simulink model "DDMRsimulink"  (R2018a)
settings: Solver=VariableStepAuto  StartTime=0.0  StopTime=tf  FixedStep=5e-3  RelTol=1e-3
InitFcn:
  | run('DDMRsimulinkParameters.m')
values from neighbouring files (symbols this model uses):
  d = 0.0445    [DDMRsimulinkParameters.m]    (also in Params.m = 1; dataSimulink.mat; p3dx_constants.m = 0.381)
  J = M*1.2e-1    (= 1.08)    [DDMRsimulinkParameters.m]    (also in Params.m = 1; dataSimulink.mat = 0.192; p3dx_constants.m = 0.2641395)
  Kb = 0.023    [DDMRsimulinkParameters.m]    (also in Params.m = 1; dataSimulink.mat = 0.029; p3dx_constants.m = 0.08)
  Kt = 0.029    [DDMRsimulinkParameters.m]    (also in Params.m = 1; dataSimulink.mat = 0.023; p3dx_constants.m = 0.01)
  L = 0.1655    [DDMRsimulinkParameters.m]    (also in Params.m = 1; dataSimulink.mat; p3dx_constants.m = 0.381)
  La = 0.66e-3    (= 0.00066)    [DDMRsimulinkParameters.m]    (also in Params.m = 1; dataSimulink.mat; p3dx_constants.m = 0.1)
  M = 9    [DDMRsimulinkParameters.m]    (also in Params.m = 1; dataSimulink.mat = 1.6; p3dx_constants.m)
  N = 38.3    [DDMRsimulinkParameters.m]    (also in Params.m = 1; dataSimulink.mat = 1; p3dx_constants.m = 38.1)
  R = 195e-3/2    (= 0.0975)    [DDMRsimulinkParameters.m]    (also in Params.m = 1; dataSimulink.mat = 0.097541; p3dx_constants.m)
  Ra = 0.71    [DDMRsimulinkParameters.m]    (also in Params.m = 1; dataSimulink.mat; p3dx_constants.m = 1)
  vaL = 5    [ExecutarSimulacoesP3DX.m]
  vaR = 12    [ExecutarSimulacoesP3DX.m]
settings Model: Creator=Egydio Tadeu  LastModifiedBy=Egydio Tadeu

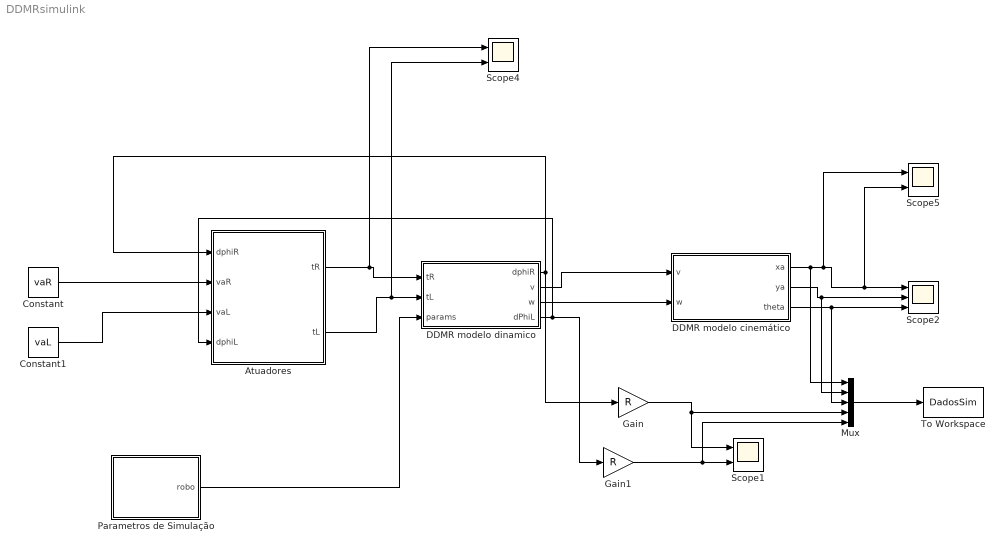
== system DDMRsimulink ==
  Atuadores : Subsystem
  Constant : Constant  Value=vaR
  Constant1 : Constant  Value=vaL
  DDMR modelo cinemático : Subsystem
  DDMR modelo dinamico : Subsystem
  Gain : Gain  Gain=R
  Gain1 : Gain  Gain=R
  Mux : Mux  Inputs=5
  Parametros de Simulação : Subsystem
  Scope1 : Scope  NumInputPorts=2
  Scope2 : Scope  NumInputPorts=3
  Scope4 : Scope  NumInputPorts=2
  Scope5 : Scope  NumInputPorts=2
  To Workspace : ToWorkspace  VariableName=DadosSim  SaveFormat=Structure With Time  SampleTime=-1
  wires:
  Parametros de Simulação/1(robo) -> DDMR modelo dinamico/3(params)
  Atuadores/1(tR) -> Scope4/1, DDMR modelo dinamico/1(tR)
  Atuadores/2(tL) -> Scope4/2, DDMR modelo dinamico/2(tL)
  DDMR modelo dinamico/4(dPhiL) -> Gain1/1, Atuadores/4(dphiL)
  DDMR modelo dinamico/1(dphiR) -> Atuadores/1(dphiR), Gain/1
  Gain1/1 -> Mux/5, Scope1/2
  Gain/1 -> Mux/4, Scope1/1
  DDMR modelo dinamico/2(v) -> DDMR modelo cinemático/1(v)
  DDMR modelo dinamico/3(w) -> DDMR modelo cinemático/2(w)
  DDMR modelo cinemático/2(ya) -> Mux/2, Scope2/2
  DDMR modelo cinemático/3(theta) -> Mux/3, Scope2/3
  DDMR modelo cinemático/1(xa) -> Mux/1, Scope5/1, Scope5/2, Scope2/1
  Constant/1 -> Atuadores/2(vaR)
  Constant1/1 -> Atuadores/3(vaL)
  Mux/1 -> To Workspace/1

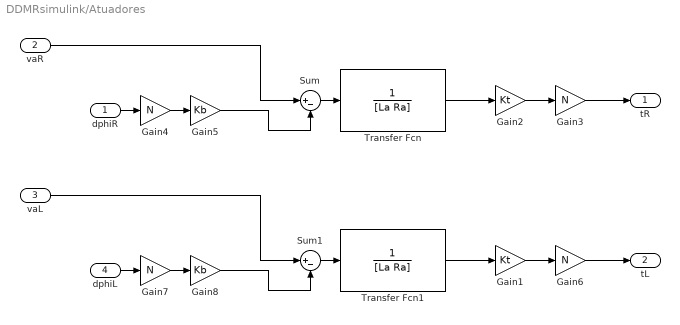
== system DDMRsimulink/Atuadores ==
  dphiR : Inport
  vaR : Inport  Port=2
  vaL : Inport  Port=3
  dphiL : Inport  Port=4
  Gain1 : Gain  Gain=Kt
  Gain2 : Gain  Gain=Kt
  Gain{3..4,6..7} (4 alike) : Gain  Gain=N
  Gain5 : Gain  Gain=Kb
  Gain8 : Gain  Gain=Kb
  Sum : Sum  Inputs=|+-
  Sum1 : Sum  Inputs=|+-
  Transfer Fcn : TransferFcn  Denominator=[La Ra]
  Transfer Fcn1 : TransferFcn  Denominator=[La Ra]
  tR : Outport
  tL : Outport  Port=2
  wires:
  Gain3/1 -> tR/1
  Transfer Fcn/1 -> Gain2/1
  Gain2/1 -> Gain3/1
  vaR/1 -> Sum/1
  Gain4/1 -> Gain5/1
  dphiR/1 -> Gain4/1
  Gain5/1 -> Sum/2
  dphiL/1 -> Gain7/1
  Gain6/1 -> tL/1
  Gain1/1 -> Gain6/1
  Transfer Fcn1/1 -> Gain1/1
  Gain7/1 -> Gain8/1
  Gain8/1 -> Sum1/2
  Sum/1 -> Transfer Fcn/1
  Sum1/1 -> Transfer Fcn1/1
  vaL/1 -> Sum1/1

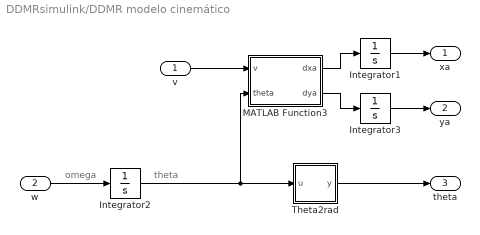
== system DDMRsimulink/DDMR modelo cinemático ==
  note: theta
  note: omega
  v : Inport
  w : Inport  Port=2
  Integrator1 : Integrator
  Integrator2 : Integrator
  Integrator3 : Integrator
  MATLAB Function3 : MATLAB Function  TreatAsAtomicUnit=on
  Theta2rad : MATLAB Function  TreatAsAtomicUnit=on
  xa : Outport
  ya : Outport  Port=2
  theta : Outport  Port=3
  wires:
  w/1 -> Integrator2/1
  v/1 -> MATLAB Function3/1(v)
  MATLAB Function3/1(dxa) -> Integrator1/1
  MATLAB Function3/2(dya) -> Integrator3/1
  Integrator1/1 -> xa/1
  Integrator3/1 -> ya/1
  Integrator2/1 -> MATLAB Function3/2(theta), Theta2rad/1(u)
  Theta2rad/1(y) -> theta/1

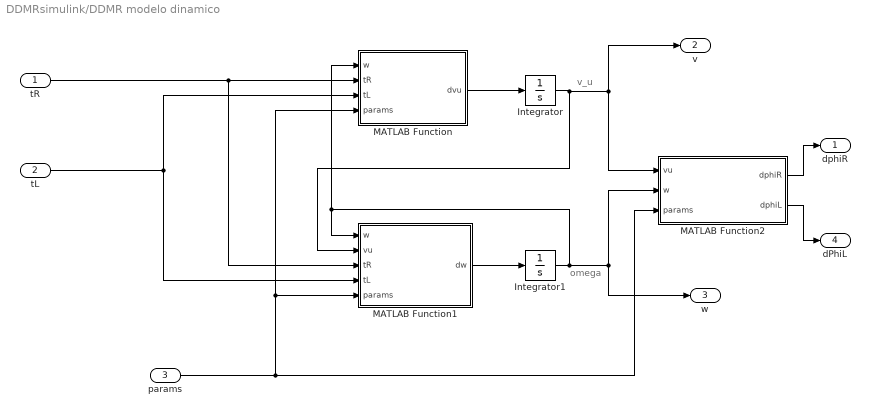
== system DDMRsimulink/DDMR modelo dinamico ==
  note: omega
  note: v_u
  tR : Inport
  tL : Inport  Port=2
  params : Inport  Port=3
  Integrator : Integrator
  Integrator1 : Integrator
  MATLAB Function : MATLAB Function  TreatAsAtomicUnit=on
  MATLAB Function1 : MATLAB Function  TreatAsAtomicUnit=on
  MATLAB Function2 : MATLAB Function  TreatAsAtomicUnit=on
  dphiR : Outport
  v : Outport  Port=2
  w : Outport  Port=3
  dPhiL : Outport  Port=4
  wires:
  Integrator/1 -> v/1, MATLAB Function2/1(vu), MATLAB Function1/2(vu)
  Integrator1/1 -> MATLAB Function/1(w), MATLAB Function1/1(w), w/1, MATLAB Function2/2(w)
  MATLAB Function2/1(dphiR) -> dphiR/1
  MATLAB Function/1(dvu) -> Integrator/1
  params/1 -> MATLAB Function2/3(params), MATLAB Function1/5(params), MATLAB Function/4(params)
  MATLAB Function1/1(dw) -> Integrator1/1
  tR/1 -> MATLAB Function1/3(tR), MATLAB Function/2(tR)
  tL/1 -> MATLAB Function1/4(tL), MATLAB Function/3(tL)
  MATLAB Function2/2(dphiL) -> dPhiL/1

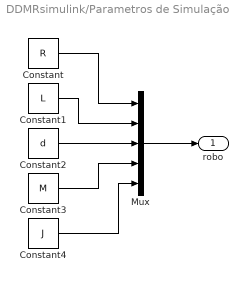
== system DDMRsimulink/Parametros de Simulação ==
  Constant : Constant  Value=R
  Constant1 : Constant  Value=L
  Constant2 : Constant  Value=d
  Constant3 : Constant  Value=M
  Constant4 : Constant  Value=J
  Mux : Mux  Inputs=5
  robo : Outport
  wires:
  Constant/1 -> Mux/1
  Mux/1 -> robo/1
  Constant2/1 -> Mux/3
  Constant3/1 -> Mux/4
  Constant4/1 -> Mux/5
  Constant1/1 -> Mux/2

== matlab function DDMRsimulink/DDMR modelo dinamico/MATLAB Function1 ==
  data: w input; dw output; vu input; tR input; tL input; params input
function dw = fcn(w, vu, tR, tL, params)

R = params(1);
L = params(2);
d = params(3);
M = params(4);
J = params(5);

dw = L*(tR-tL)/(R*(M*d*d + J)) - w*vu*M*d/(M*d*d + J);

== matlab function DDMRsimulink/DDMR modelo dinamico/MATLAB Function ==
  data: w input; dvu output; tR input; tL input; params input
function dvu = fcn(w, tR, tL, params)

R = params(1);
d = params(3);
M = params(4);

dvu = (tR+tL)/(M*R) + d*w*w;

== matlab function DDMRsimulink/DDMR modelo dinamico/MATLAB Function2 ==
  data: vu input; dphiR output; w input; params input; dphiL output
function [dphiR, dphiL] = fcn(vu, w, params)

R = params(1);
L = params(2);

dphiR = (vu+L*w)/R;
dphiL = (vu-L*w)/R;

end

== matlab function DDMRsimulink/DDMR modelo cinemático/Theta2rad ==
  data: u input; y output
function y = fcn(u)

y = u;
while (abs(y) > pi)
    if(y > 0)
        y = y - 2*pi;
    else
        y = y + 2*pi;
    end
end

end

== matlab function DDMRsimulink/DDMR modelo cinemático/MATLAB Function3 ==
  data: v input; dxa output; theta input; dya output
function [dxa, dya]  = fcn(v, theta)

dxa = cos(theta)*v;
dya = sin(theta)*v;
